simulink subsystem "WB_update"  (R2021b)
settings: Solver=VariableStepAuto  StartTime=0.0  StopTime=10.0  RelTol=1e-3
settings Model: Creator=bogru  LastModifiedBy=bogru

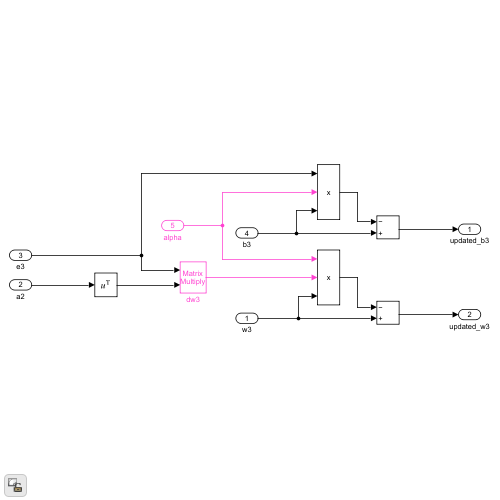
[thumbnail: Simulink's stored preview of the top-level diagram]
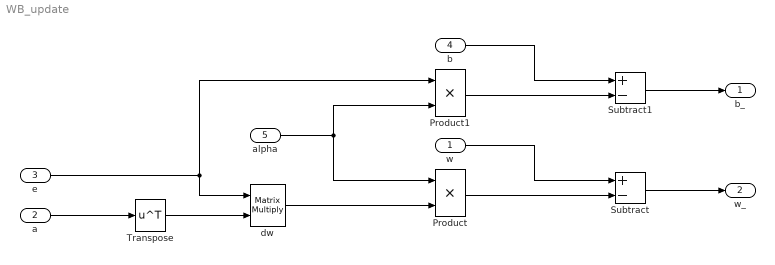
== system WB_update ==
  w : Inport
  a : Inport  Port=2
  e : Inport  Port=3
  b : Inport  Port=4
  alpha : Inport  Port=5
  Product : Product
  Product1 : Product
  Subtract : Sum  Inputs=+-
  Subtract1 : Sum  Inputs=+-
  Transpose : Math  Operator=transpose  SaturateOnIntegerOverflow=on
  dw : Product  Multiplication=Matrix(*)
  b_ : Outport
  w_ : Outport  Port=2
  wires:
  e/1 -> dw/1, Product1/1
  Transpose/1 -> dw/2
  a/1 -> Transpose/1
  alpha/1 -> Product/1, Product1/2
  Subtract/1 -> w_/1
  Subtract1/1 -> b_/1
  dw/1 -> Product/2
  w/1 -> Subtract/1
  Product1/1 -> Subtract1/2
  b/1 -> Subtract1/1
  Product/1 -> Subtract/2
